simulink model "D_20231120_Modell_Inbetriebnahme_BreakOutBox_Jetson"  (R2022b)
settings: Solver=ode1  StartTime=0.0  StopTime=inf  FixedStep=Ts  RelTol=1e-3
PreLoadFcn:
  | pulsePeriod = 0.05;
  | 
  | Ts = 0.001;
  | 
  | FPGA_Frequency = 75000000;
  | 
  | ts_IO691 = 5e-3;
PostLoadFcn:
  | ewolfSetUp
InitFcn:
  | pulsePeriod = 0.05;
  | 
  | Ts = 0.001;
  | 
  | FPGA_Frequency = 75000000;
  | 
  | ts_IO691 = 5e-3;
StopFcn:
  | Simulink.sdi.clearPreferences;
  | if isfile(['sdi_view_',bdroot,'.mldatx'])
  | Simulink.sdi.view;
  | pause(3);
  | Simulink.sdi.loadView(['sdi_view_',bdroot,]);
  | end
model workspace (MAT data in the model file):
  MaxDreh = 1
values from neighbouring files (symbols this model uses):
  max_ac = 2    [ewolfSetUp.m]
  min_ac = -3    [ewolfSetUp.m]
  PredictionHorizon = 30    [ewolfSetUp.m]
undefined symbols (not defined in the file or in its folder): canChannel, DiscIntNeverNeededParam, Ended, HS, IO291, IO397, max_steer_car, min_steer_car, sigbuilder_block, Single
libraries: lllalib x255, canmsglib x146, simulink x42, speedgoatlib_IO191 x5, speedgoatlib_IO291 x5, slrealtimeiplib x3, speedgoatlib_IO691 x3, slrealtimeutilitieslib x2, spsEdgeDetectorLib x1, simulink_extras x1, speedgoatlib_fpga_dio x1, speedgoatlib_fpga_quadrature x1
(part 1 of 8)
settings Model: SimulationMode=external  ExtModeEnableFloating=off  Creator=daniel.carretero  LastModifiedBy=admin
settings SolverCC: ConcurrentTasks=on  PositivePriorityOrder=on  AutoInsertRateTranBlk=on
settings DataIOCC: ReturnWorkspaceOutputs=off
settings OptimizationCC: BlockReduction=off  OptimizeBlockIOStorage=off
settings DebuggingCC: TasksWithSamePriorityMsg=none  ParameterPrecisionLossMsg=none
settings HardwareCC: ProdBitPerLong=64  ProdLongLongMode=on  ProdHWDeviceType=Intel->x86-64 (Linux 64)
settings ModelReferenceCC: EnableRefExpFcnMdlSchedulingChecks=on
settings RTWCC: Description=Simulink Real-Time  SystemTargetFile=slrealtime.tlc  TemplateMakefile=slrealtime_default_tmf  RTWVerbose=off  Toolchain=Simulink Real-Time Toolchain  BuildConfiguration=Faster Runs  CodeExecutionProfiling=on  TargetLang=C++  DLArmComputeVersion=19.05

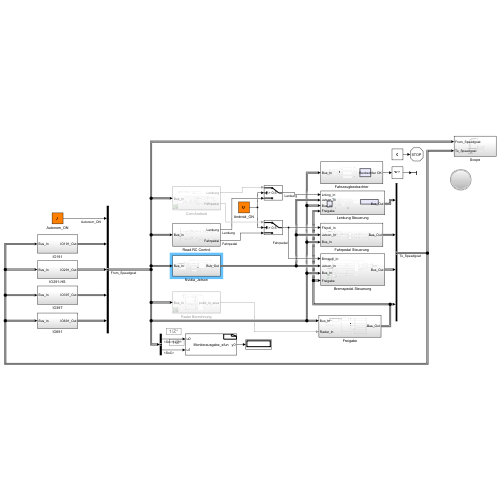
[thumbnail: Simulink's stored preview of the top-level diagram]
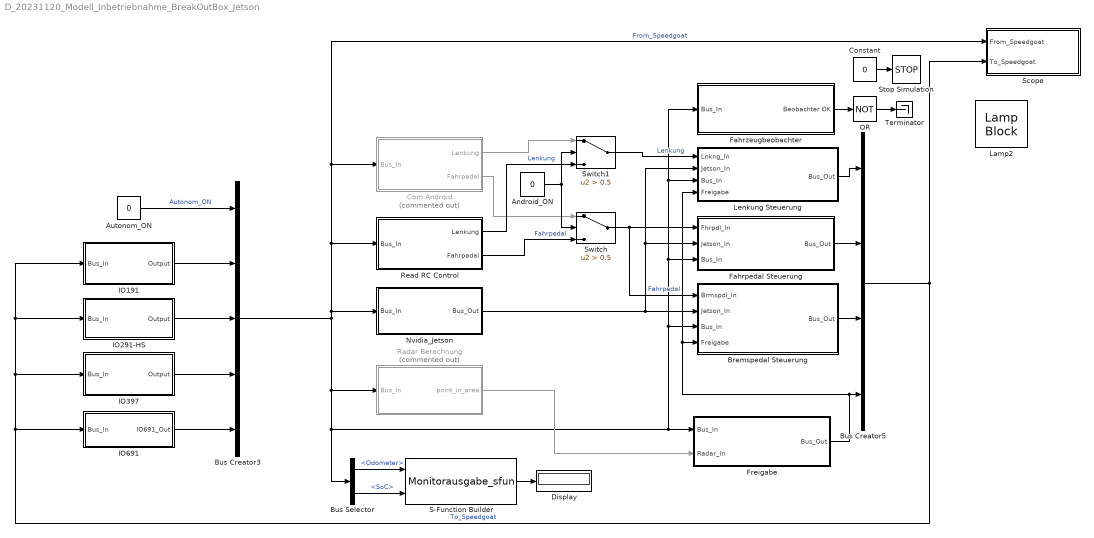
== system D_20231120_Modell_Inbetriebnahme_BreakOutBox_Jetson ==
  Android_ON : Constant  Value=0
  Autonom_ON : Constant  Value=0
  Bremspedal Steuerung : Subsystem
  Bus Creator3 : BusCreator  Inputs=5
  Bus Creator5 : BusCreator  Inputs=4
  Bus Selector : BusSelector  OutputSignals=IO691_Out.IO691_CAN_eWolf.Odometer,IO691_Out.IO691_CAN_eWolf.SoC
  Com Android : Subsystem  Commented=on
  Constant : Constant  Value=0
  Display : Display
  Fahrpedal Steuerung : Subsystem
  Fahrzeugbeobachter : Subsystem
  Freigabe : Subsystem
  IO191 : Subsystem
  IO291-HS : Subsystem
  IO397 : Subsystem
  IO691 : Subsystem
  Lamp2 : LampBlock  LabelPosition=Hide
  Lenkung Steuerung : Subsystem
  Nvidia_Jetson : Subsystem
  OR : Logic  Operator=NOT  AllPortsSameDT=off  OutDataTypeStr=boolean
  Radar Berechnung : Subsystem  Description=|  Commented=on
      | Extract radar data from CAN messages and create vector object with: 1788 fields:
      | 
      | 1. Timestamp
      | 2. cycle_count
      | 3. number of Objects
      | 4. radar timestamp_header
      | 5. CAN ID
      | +++++++++++++++++++++
      | % last point
      | 6. range
      | 7. az
      | 8. vr
      | 9. rcs
      | 10. el
      | ----------------------------------
      | % last point -1
      | 11. range
      | 12. az
      | 13. vr
      | 14. rcs
      | 15. el
      |  ...
      | 
      | empty points, all values == 0
  Read RC Control : Subsystem
  S-Function Builder : S-Function  FunctionName=Monitorausgabe_sfun  SFunctionModules=Monitorausgabe_sfun_wrapper.cpp  SFunctionDeploymentMode=off  EnableBusSupport=off  mask(S-Function Builder){}
      mask help: Simulink:masks:SFunctionBuilder_MD
      mask init:
      | val = [[.9  0.75 0.75 1 1 .9 .9 1]',[1 1 0.75 0.75 .9 .9 1 .9]'];try , sys = get_param(gcb,'SfunBuilderFcnName');if isempty(sys), sys = get_param(gcb,'FunctionName'); end,catch, sys = get_param(gcb,'FunctionName'); end
      settings: CopyFcn=set_param(gcbh,'LinkStatus','none')  OpenFcn=sfunctionwizard(gcbh)
      mask Display: plot(val(:,1),val(:,2)),disp(sys),port_label('input',1,'u0'),port_label('input',2,'u1'),port_label('output',1,'y0')
  Scope : Subsystem
  Stop Simulation : Stop
  Switch : Switch  Criteria=u2 > Threshold  Threshold=0.5  SaturateOnIntegerOverflow=off  InputSameDT=off
  Switch1 : Switch  Criteria=u2 > Threshold  Threshold=0.5  SaturateOnIntegerOverflow=off  InputSameDT=off
  Terminator : Terminator
  wires:
  IO191/1(Output) -> Bus Creator3/2
  IO291-HS/1(Output) -> Bus Creator3/3
  IO397/1(Output) -> Bus Creator3/4
  Bus Creator3/1 -> Scope/1(From_Speedgoat), Com Android/1(Bus_In), Read RC Control/1(Bus_In), Nvidia_Jetson/1(Bus_In), Radar Berechnung/1(Bus_In), Bus Selector/1, Bremspedal Steuerung/3(Bus_In), Fahrzeugbeobachter/1(Bus_In), Lenkung Steuerung/3(Bus_In), Fahrpedal Steuerung/3(Bus_In), Freigabe/1(Bus_In)  "From_Speedgoat"
  Switch/1 -> Bremspedal Steuerung/1(Brmspdl_In), Fahrpedal Steuerung/1(Fhrpdl_In)  "Fahrpedal"
  IO691/1(IO691_Out) -> Bus Creator3/5
  Fahrpedal Steuerung/1(Bus_Out) -> Bus Creator5/2
  Freigabe/1(Bus_Out) -> Bus Creator5/4, Lenkung Steuerung/4(Freigabe), Bremspedal Steuerung/4(Freigabe)
  Bremspedal Steuerung/1(Bus_Out) -> Bus Creator5/3
  Bus Creator5/1 -> IO191/1(Bus_In), IO291-HS/1(Bus_In), IO397/1(Bus_In), IO691/1(Bus_In), Scope/2(To_Speedgoat)  "To_Speedgoat"
  Nvidia_Jetson/1(Bus_Out) -> Bremspedal Steuerung/2(Jetson_In), Lenkung Steuerung/2(Jetson_In), Fahrpedal Steuerung/2(Jetson_In)
  Autonom_ON/1 -> Bus Creator3/1  "Autonom_ON"
  Radar Berechnung/1(point_in_area) -> Freigabe/2(Radar_In)
  Bus Selector/1 -> S-Function Builder/1  "<Odometer>"
  S-Function Builder/1 -> Display/1
  Bus Selector/2 -> S-Function Builder/2  "<SoC>"
  Com Android/1(Lenkung) -> Switch1/1
  Com Android/2(Fahrpedal) -> Switch/1
  Read RC Control/1(Lenkung) -> Switch1/3  "Lenkung"
  Read RC Control/2(Fahrpedal) -> Switch/3  "Fahrpedal"
  Android_ON/1 -> Switch1/2, Switch/2
  Constant/1 -> Stop Simulation/1
  Fahrzeugbeobachter/1(Beobachter OK) -> OR/1
  OR/1 -> Terminator/1
  Switch1/1 -> Lenkung Steuerung/1(Lnkng_In)  "Lenkung"
  Lenkung Steuerung/1(Bus_Out) -> Bus Creator5/1

== system D_20231120_Modell_Inbetriebnahme_BreakOutBox_Jetson/Bremspedal Steuerung ==
  Brmspdl_In : Inport
  Jetson_In : Inport  Port=2
  Bus_In : Inport  Port=3
  Freigabe : Inport  Port=4
  1-D Lookup Table2 : Lookup_n-D  NumberOfTableDimensions=1  BreakpointsForDimension1=[min_ac max_ac]  Table=[-1 1]  InternalRulePriority=Speed  RndMeth=Simplest
  AND3 : Logic  AllPortsSameDT=off  OutDataTypeStr=boolean
  AND4 : Logic  AllPortsSameDT=off  OutDataTypeStr=boolean
  Bus Creator : BusCreator  Inputs=2
  Bus Selector : BusSelector  OutputSignals=IO397_Out.IO397_DIO.IO397_DI_Ch8_Bremsaktuator_Hall_1,IO397_Out.IO397_DIO.IO397_DI_Ch9_Bremsaktuator_Hall_2,IO291_Out.IO291_Iso_DI.IO291_DI_CH3_Brmslcht,IO397_Out.IO397_QAD.IO397_QAD_Turns,Autonom_ON
  Bus Selector1 : BusSelector  OutputSignals=acceleration
  Bus Selector2 : BusSelector  OutputSignals=Taster_Freigabe
  Gain -1 : Gain  Gain=-1
  Moving Average : Subsystem
  Moving Average1 : Subsystem
  QAD Steuerung : Subsystem  Commented=on
  QAD Steuerung1 : Subsystem
  Saturation3 : Saturate  UpperLimit=0  LowerLimit=-1
  Switch : Switch  Criteria=u2 > Threshold  Threshold=0.5  SaturateOnIntegerOverflow=off  InputSameDT=off
  Bus_Out : Outport
  wires:
  Brmspdl_In/1 -> Switch/3
  Saturation3/1 -> Gain -1/1
  Bus_In/1 -> Bus Selector/1
  AND3/1 -> Bus Creator/1  "Bremsaktuator_1"
  AND4/1 -> Bus Creator/2  "Bremsaktuator_2"
  Bus Selector/4 -> QAD Steuerung/1(<QAD_Turns>)  "<IO397_QAD_Turns>"
  Gain -1/1 -> QAD Steuerung1/4(Brk), QAD Steuerung/2(u)  "Bremssignal"
  Bus Selector/1 -> Moving Average/1(In)  "<IO397_DI_Ch8_Bremsaktuator_Hall_1>"
  Bus Selector/2 -> Moving Average1/1(In)  "<IO397_DI_Ch9_Bremsaktuator_Hall_2>"
  Moving Average/1(Hall_A) -> QAD Steuerung1/1(Hall_A)  "Hall_A"
  Moving Average1/1(Hall_B) -> QAD Steuerung1/2(Hall_B)  "Hall_B"
  QAD Steuerung1/1(Rel_1) -> AND3/2  "Rel_1"
  QAD Steuerung1/2(Rel_2) -> AND4/2  "Rel_2"
  Bus Creator/1 -> Bus_Out/1  "Brmskttr"
  Jetson_In/1 -> Bus Selector1/1
  Bus Selector1/1 -> 1-D Lookup Table2/1  "<acceleration>"
  Bus Selector/5 -> Switch/2  "<Autonom_ON>"
  Switch/1 -> Saturation3/1
  1-D Lookup Table2/1 -> Switch/1
  Bus Selector/3 -> QAD Steuerung1/3(BrkPdlSwtch)  "<IO291_DI_CH3_Brmslcht>"
  Freigabe/1 -> Bus Selector2/1
  Bus Selector2/1 -> AND4/1, AND3/1  "<Taster_Freigabe>"

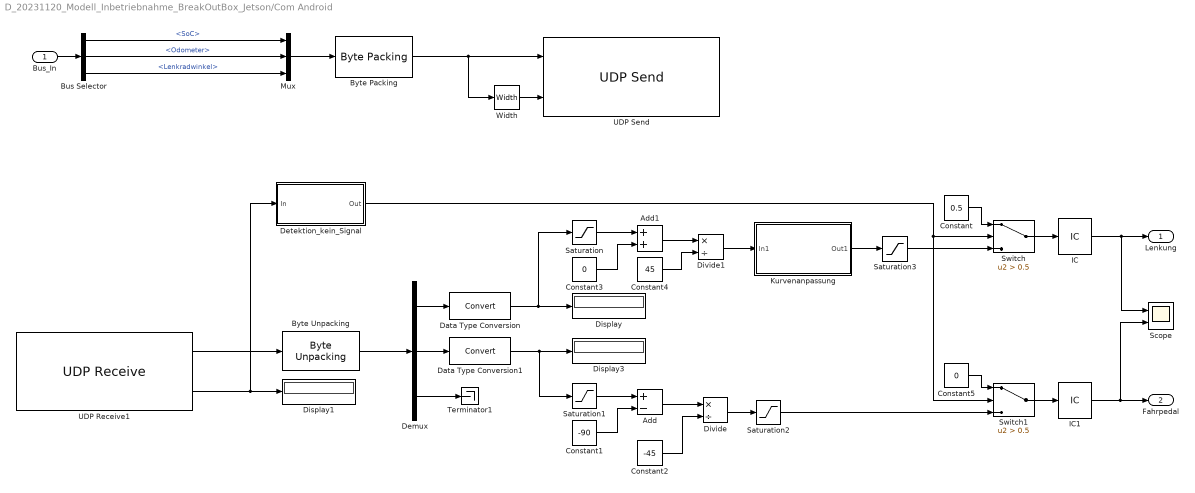
== system D_20231120_Modell_Inbetriebnahme_BreakOutBox_Jetson/Com Android ==
  Bus_In : Inport
  Add : Sum  Inputs=+-
  Add1 : Sum
  Bus Selector : BusSelector  OutputSignals=IO691_Out.IO691_CAN_eWolf.SoC,IO691_Out.IO691_CAN_eWolf.Odometer,IO691_Out.IO691_CAN_Sensoren.Lenkradwinkel
  Byte Packing : slrealtimeutilitieslib/Byte Packing  MaskPackedDataType=uint8  MaskUnpackedDataTypes={'double'}  MaskAlignment=1
  Byte Unpacking : slrealtimeutilitieslib/Byte Unpacking  MaskUnpackedDataTypes={'single'}  MaskUnpackedDataSizes={[3]}  MaskAlignment=1
  Constant : Constant  Value=0.5
  Constant1 : Constant  Value=-90
  Constant2 : Constant  Value=-45
  Constant3 : Constant  Value=0
  Constant4 : Constant  Value=45
  Constant5 : Constant  Value=0
  Data Type Conversion : DataTypeConversion  SaturateOnIntegerOverflow=off  RndMeth=Floor
  Data Type Conversion1 : DataTypeConversion  SaturateOnIntegerOverflow=off  RndMeth=Floor
  Demux : Demux  Outputs=3
  Detektion_kein_Signal : Subsystem
  Display : Display
  Display1 : Display
  Display3 : Display
  Divide : Product  Inputs=*/
  Divide1 : Product  Inputs=*/
  IC : InitialCondition  Value=0.5
  IC1 : InitialCondition  Value=0
  Kurvenanpassung : Subsystem
  Mux : Mux  Inputs=3
  Saturation : Saturate  UpperLimit=45  LowerLimit=-45
  Saturation1 : Saturate  UpperLimit=-45  LowerLimit=-135
  Saturation2 : Saturate  UpperLimit=1  LowerLimit=-1
  Saturation3 : Saturate  UpperLimit=1  LowerLimit=-1
  Scope : Scope  NumInputPorts=2
  Switch : Switch  Criteria=u2 > Threshold  Threshold=0.5  SaturateOnIntegerOverflow=off  InputSameDT=off
  Switch1 : Switch  Criteria=u2 > Threshold  Threshold=0.5  SaturateOnIntegerOverflow=off  InputSameDT=off
  Terminator1 : Terminator
  UDP Receive1 : slrealtimeiplib/UDP Receive  useHostTargetConn=off  ipAddress=192.168.9.10  localPort=25001  rcvWidth=12  rcvFmAny=on  fmAddress='10.10.10.10'  sampleTime=0.001  enableMessage=off  maxPackets=1
  UDP Send : slrealtimeiplib/UDP Send  useHostTargetConn=off  toAddress='192.168.9.255'  toPort=25000  sampleTime=0.1  enableMessage=off  ipAddress=192.168.9.10  localPort=25000
  Width : Width
  Lenkung : Outport
  Fahrpedal : Outport  Port=2
  wires:
  Demux/2 -> Data Type Conversion1/1
  Width/1 -> UDP Send/2
  Byte Unpacking/1 -> Demux/1
  Byte Packing/1 -> Width/1, UDP Send/1
  Bus Selector/2 -> Mux/2  "<Odometer>"
  UDP Receive1/1 -> Byte Unpacking/1
  Mux/1 -> Byte Packing/1
  Demux/3 -> Terminator1/1
  Bus Selector/1 -> Mux/1  "<SoC>"
  Demux/1 -> Data Type Conversion/1
  UDP Receive1/2 -> Detektion_kein_Signal/1(In), Display1/1
  Data Type Conversion1/1 -> Saturation1/1, Display3/1
  Data Type Conversion/1 -> Saturation/1, Display/1
  Bus_In/1 -> Bus Selector/1
  Bus Selector/3 -> Mux/3  "<Lenkradwinkel>"
  Saturation1/1 -> Add/1
  Constant1/1 -> Add/2
  Add/1 -> Divide/1
  Constant2/1 -> Divide/2
  Divide/1 -> Saturation2/1
  Saturation2/1 -> Switch1/3
  Saturation/1 -> Add1/1
  Constant3/1 -> Add1/2
  Add1/1 -> Divide1/1
  Constant4/1 -> Divide1/2
  IC/1 -> Scope/1, Lenkung/1
  IC1/1 -> Scope/2, Fahrpedal/1
  Divide1/1 -> Kurvenanpassung/1(In1)
  Switch/1 -> IC/1
  Switch1/1 -> IC1/1
  Detektion_kein_Signal/1(Out) -> Switch1/2, Switch/2
  Constant/1 -> Switch/1
  Constant5/1 -> Switch1/1
  Saturation3/1 -> Switch/3
  Kurvenanpassung/1(Out1) -> Saturation3/1

== system D_20231120_Modell_Inbetriebnahme_BreakOutBox_Jetson/Fahrpedal Steuerung ==
  Fhrpdl_In : Inport
  Jetson_In : Inport  Port=2
  Bus_In : Inport  Port=3
  1-D Lookup Table : Lookup_n-D  NumberOfTableDimensions=1  BreakpointsForDimension1=[0:1]  Table=[0.8 4.8]  InternalRulePriority=Speed  RndMeth=Simplest
  1-D Lookup Table1 : Lookup_n-D  NumberOfTableDimensions=1  BreakpointsForDimension1=[0:1]  Table=[0.4 2.4]  InternalRulePriority=Speed  RndMeth=Simplest
  1-D Lookup Table2 : Lookup_n-D  NumberOfTableDimensions=1  BreakpointsForDimension1=[min_ac max_ac]  Table=[-1 1]  InternalRulePriority=Speed  RndMeth=Simplest
  Bias1 : Bias  SaturateOnIntegerOverflow=off
  Bias2 : Bias  SaturateOnIntegerOverflow=off
  Bus Creator : BusCreator  Inputs=2
  Bus Selector : BusSelector  OutputSignals=acceleration
  Bus Selector1 : BusSelector  OutputSignals=Autonom_ON
  IC2 : InitialCondition  Value=0.8
  IC3 : InitialCondition  Value=0.4
  Saturation3 : Saturate  UpperLimit=1  LowerLimit=0
  Switch : Switch  Criteria=u2 > Threshold  Threshold=0.5  SaturateOnIntegerOverflow=off  InputSameDT=off
  Bus_Out : Outport
  wires:
  Bias1/1 -> Bus Creator/1  "Ausgabe_Gaspedal_FP_1_G"
  Bias2/1 -> Bus Creator/2  "Ausgabe_Gaspedal_FP_2_G"
  IC2/1 -> Bias1/1
  IC3/1 -> Bias2/1
  1-D Lookup Table/1 -> IC2/1
  Saturation3/1 -> 1-D Lookup Table1/1, 1-D Lookup Table/1
  1-D Lookup Table1/1 -> IC3/1
  Bus Creator/1 -> Bus_Out/1  "Fhrpdl"
  Jetson_In/1 -> Bus Selector/1
  Bus Selector/1 -> 1-D Lookup Table2/1  "<acceleration>"
  Bus_In/1 -> Bus Selector1/1
  Bus Selector1/1 -> Switch/2  "<Autonom_ON>"
  Fhrpdl_In/1 -> Switch/3
  Switch/1 -> Saturation3/1
  1-D Lookup Table2/1 -> Switch/1

== system D_20231120_Modell_Inbetriebnahme_BreakOutBox_Jetson/Fahrzeugbeobachter ==
  note: Aukustische und optische Übergabe
      | an Fahrer
  Bus_In : Inport
  AND : Logic  Inputs=3  AllPortsSameDT=off  OutDataTypeStr=boolean
  Bus Selector : BusSelector  OutputSignals=IO691_Out.IO691_CAN_Sensoren.Lenkradwinkel,IO691_Out.IO691_CAN_eWolf.CarSpeed,IO691_Out.IO691_CAN_Sensoren.Gierrate,IO691_Out.IO691_CAN_Sensoren.Gierbeschleunigung,IO691_Out.IO691_CAN_Sensoren.AY,IO691_Out.IO691_CAN_Sensoren.AX
  Constant3 : Constant  Value=10
  Derivative : Derivative
  Fahrzeuggeschwindigkeit : MATLAB Function  TreatAsAtomicUnit=on
  IC2 : InitialCondition
  Lamp{1..4} (4 alike) : LampBlock  LabelPosition=Hide
  Lenkradwinkel : MATLAB Function  TreatAsAtomicUnit=on
  Lenkradwinkelgeschwindigkeit : MATLAB Function  TreatAsAtomicUnit=on
  Product : Product
  Terminator3 : Terminator  Commented=on
  Terminator4 : Terminator
  Terminator5 : Terminator  Commented=on
  Terminator6 : Terminator  Commented=on
  Beobachter OK : Outport
  wires:
  Bus_In/1 -> Bus Selector/1
  Bus Selector/3 -> Terminator4/1  "<Gierrate>"
  Bus Selector/4 -> Terminator3/1  "<Gierbeschleunigung>"
  Bus Selector/6 -> Terminator6/1  "<AX>"
  Bus Selector/5 -> Terminator5/1  "<AY>"
  Bus Selector/1 -> Derivative/1, Lenkradwinkel/2(lenkradwinkel)  "<Lenkradwinkel>"
  Constant3/1 -> Product/2
  Bus Selector/2 -> Product/1  "<CarSpeed>"
  Product/1 -> Lenkradwinkel/1(geschwindigkeitFahrzeug), Fahrzeuggeschwindigkeit/1(geschwindigkeitFahrzeug), Lenkradwinkelgeschwindigkeit/1(geschwindigkeitFahrzeug)
  Derivative/1 -> Lenkradwinkelgeschwindigkeit/2(geschwindigkeitLenkradwinkel)
  Lenkradwinkelgeschwindigkeit/1(geschwindigkeitLenkradwinkel_OK) -> AND/2
  Lenkradwinkel/1(lenkradwinkel_OK) -> AND/1
  Fahrzeuggeschwindigkeit/1(geschwindigkeitFahrzeug_OK) -> AND/3
  AND/1 -> IC2/1
  IC2/1 -> Beobachter OK/1

== system D_20231120_Modell_Inbetriebnahme_BreakOutBox_Jetson/Freigabe ==
  Bus_In : Inport
  Radar_In : Inport  Port=2
  Bus Creator : BusCreator  Inputs=8
  Constant13 : Constant
  Constant8 : Constant  Value=0
  Freigabe : Subsystem
  Gain{4..9} (6 alike) : Gain
  Terminator : Terminator
  Totmann : Subsystem
  Bus_Out : Outport
  wires:
  Totmann/1(Totmann_Freigabe) -> Freigabe/2(Totmann_In)
  Bus_In/1 -> Freigabe/1(Bus_In), Totmann/1(Bus_In)
  Totmann/2(Totmann_LED) -> Gain4/1
  Gain4/1 -> Bus Creator/7  "LED_Totmann"
  Gain8/1 -> Bus Creator/3  "LG_FET_1_On"
  Gain9/1 -> Bus Creator/4  "LG_FET_2_On"
  Gain7/1 -> Bus Creator/2  "FP_FET_2_On"
  Gain5/1 -> Bus Creator/6  "Taster_Freigabe"
  Freigabe/1(Freigabe_Out) -> Gain5/1, Gain9/1, Gain8/1, Gain7/1, Gain6/1
  Constant8/1 -> Bus Creator/5  "Br_Licht_On"
  Gain6/1 -> Bus Creator/1  "FP_FET_1_On"
  Bus Creator/1 -> Bus_Out/1  "Freigabe"
  Constant13/1 -> Bus Creator/8  "USS_Reverse"
  Radar_In/1 -> Terminator/1

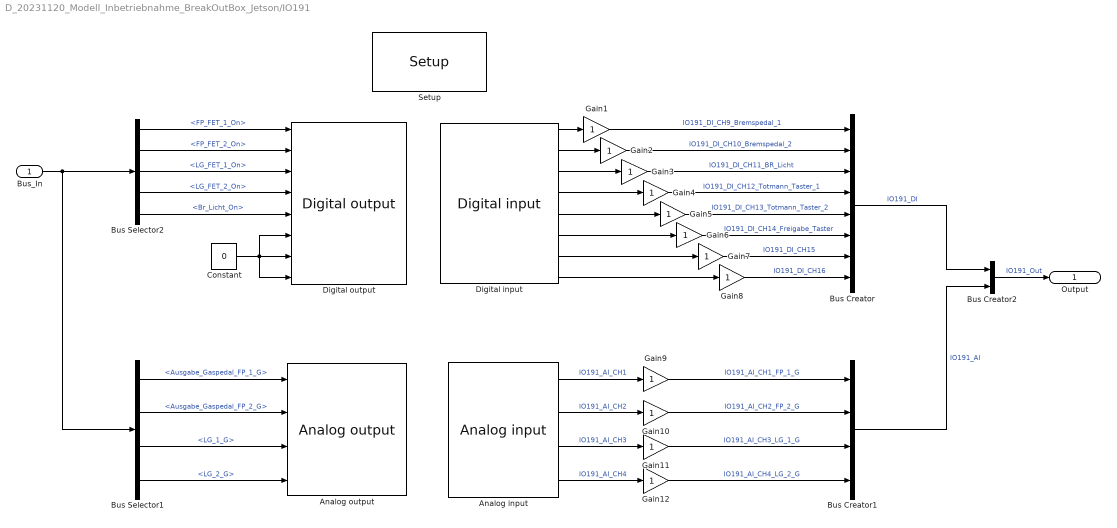
== system D_20231120_Modell_Inbetriebnahme_BreakOutBox_Jetson/IO191 ==
  Bus_In : Inport
  "Analog input " : speedgoatlib_IO191/Analog input   parModuleId=1  parSampleTime=Ts  parPciSlot=-1  parAdcChannels=[1 2 3 4]  parAdcMode=2  parAdcRanges=[4 4 4 4]  parAdcRate=100000  parAdcInitValues=[0 0]  parAdcResets=[1 1]
      settings: SourceProductName=Simulink Real-Time: Speedgoat I/O Blockset
  "Analog output " : speedgoatlib_IO191/Analog output   parModuleId=1  parSampleTime=Ts  parPciSlot=-1  parDacChannels=[1 2 3 4]  parModuleType=1  parDacRanges=[1 1 1 1]  parDacInitValues=[0 0 2.5 2.5]  parDacResets=[1 1 1 1]
      settings: SourceProductName=Simulink Real-Time: Speedgoat I/O Blockset
  Bus Creator : BusCreator  Inputs=8
  Bus Creator1 : BusCreator  Inputs=4
  Bus Creator2 : BusCreator  Inputs=2
  Bus Selector1 : BusSelector  OutputSignals=Fhrpdl.Ausgabe_Gaspedal_FP_1_G,Fhrpdl.Ausgabe_Gaspedal_FP_2_G,Lnkng.LG_1_G,Lnkng.LG_2_G
  Bus Selector2 : BusSelector  OutputSignals=Freigabe.FP_FET_1_On,Freigabe.FP_FET_2_On,Freigabe.LG_FET_1_On,Freigabe.LG_FET_2_On,Freigabe.Br_Licht_On
  Constant : Constant  Value=0
  "Digital input " : speedgoatlib_IO191/Digital input   parModuleId=1  parSampleTime=Ts  parPciSlot=-1  parDiChannels=[9 10 11 12 13 14 15 16]
      settings: SourceProductName=Simulink Real-Time: Speedgoat I/O Blockset
  "Digital output " : speedgoatlib_IO191/Digital output   parModuleId=1  parSampleTime=Ts  parPciSlot=-1  parDoChannels=[1 2 3 4 5 6 7 8]  parDoInitValues=[0 0 0 0 0 0 0 0]  parDoResets=[1 1 1 1 1 1 1 1]
      settings: SourceProductName=Simulink Real-Time: Speedgoat I/O Blockset
  Gain{1..12} (12 alike) : Gain
  "Setup " : speedgoatlib_IO191/Setup   parModuleId=1  parPciSlot=-1  parTriggerSignal=TTL  parAdcChannels=[1 2 3 4]  parAdcRanges=[4 4 4 4]  parAdcChannel1=on  parAdcChannel2=on  parAdcChannel3=on  parAdcChannel4=on  parAdcChannel5=off  parAdcChannel6=off  parAdcChannel7=off  parAdcChannel8=off  parAdcMode=Single-Ended  parAdcRate=100000  parAdcRange11=+-5.12 V  parAdcRange21=+-24.576 V  parAdcRange12=+-5.12 V  parAdcRange22=+-24.576 V  parAdcRange13=+-5.12 V  parAdcRange23=+-24.576 V  parAdcRange14=+-5.12 V  parAdcRange24=+-24.576 V  parAdcRange15=+-10.24 V  parAdcRange25=+-24.576 V  parAdcRange16=+-10.24 V  parAdcRange26=+-24.576 V  parAdcRange17=+-10.24 V  parAdcRange27=+-24.576 V  parAdcRange18=+-10.24 V  parAdcRange28=+-24.576 V  parDacChannels=[1 2 3 4]  parDacChannel1=on  parDacChannel2=on  parDacChannel3=on  parDacChannel4=on  parDacMode=Single-Ended  parDacRanges=[1 1 1 1]  parDacInitValues=[0 0 2.5 2.5]  parDacResets=[1 1 1 1]  parDacRange1=0 V to 5 V  parDacInitValue1=0  parDacReset1=on  parDacRange2=0 V to 5 V  parDacInitValue2=0  parDacReset2=on  parDacRange3=0 V to 5 V  parDacInitValue3=2.5  parDacReset3=on  parDacRange4=0 V to 5 V  parDacInitValue4=2.5  parDacReset4=on  parDiChannels=[9 10 11 12 13 14 15 16]  parDoChannels=[1 2 3 4 5 6 7 8]  parDioFirstControl=1  parDioSecondControl=0  parDioChannel1=Out  parExtra1=I  parExtra2=I  parExtra3=I  parDioChannel2=In  parDioChannel3=In  parDioChannel4=In  parDioChannel5=In  parDioChannel6=In  parDioChannel7=In  parDioChannel8=In  parDioChannel9=In  parDoInitValues=[0 0 0 0]  parDoResets=[1 1 1 1]  parDoInitValue1=0  parDoReset1=on  parDoInitValue2=0  parDoReset2=on  parDoInitValue3=0  parDoReset3=on  parDoInitValue4=0  parDoReset4=on  parDoInitValue5=0  parDoReset5=on  parDoInitValue6=0  parDoReset6=on  parDoInitValue7=0  parDoReset7=on  parDoInitValue8=0  parDoReset8=on  parDoInitValue9=0  parDoReset9=on  parDoInitValue10=0  parDoReset10=on  parDoInitValue11=0  parDoReset11=on  parDoInitValue12=0  parDoReset12=on  parDoInitValue13=0  parDoReset13=on  parDoInitValue14=0  parDoReset14=on  parDoInitValue15=0  parDoReset15=on  parDoInitValue16=0  parDoReset16=on
      settings: SourceProductName=Simulink Real-Time: Speedgoat I/O Blockset
  Output : Outport
  wires:
  "Digital input "/7 -> Gain7/1
  "Digital input "/1 -> Gain1/1
  "Digital input "/6 -> Gain6/1
  "Digital input "/8 -> Gain8/1
  "Digital input "/5 -> Gain5/1
  "Digital input "/4 -> Gain4/1
  "Digital input "/3 -> Gain3/1
  "Digital input "/2 -> Gain2/1
  Gain1/1 -> Bus Creator/1  "IO191_DI_CH9_Bremspedal_1"
  Gain2/1 -> Bus Creator/2  "IO191_DI_CH10_Bremspedal_2"
  Gain3/1 -> Bus Creator/3  "IO191_DI_CH11_BR_Licht"
  Gain4/1 -> Bus Creator/4  "IO191_DI_CH12_Totmann_Taster_1"
  Gain5/1 -> Bus Creator/5  "IO191_DI_CH13_Totmann_Taster_2"
  Gain6/1 -> Bus Creator/6  "IO191_DI_CH14_Freigabe_Taster"
  Gain7/1 -> Bus Creator/7  "IO191_DI_CH15"
  Gain8/1 -> Bus Creator/8  "IO191_DI_CH16"
  "Analog input "/1 -> Gain9/1  "IO191_AI_CH1"
  "Analog input "/2 -> Gain10/1  "IO191_AI_CH2"
  "Analog input "/3 -> Gain11/1  "IO191_AI_CH3"
  "Analog input "/4 -> Gain12/1  "IO191_AI_CH4"
  Bus Creator/1 -> Bus Creator2/1  "IO191_DI"
  Bus Creator1/1 -> Bus Creator2/2  "IO191_AI"
  Bus Creator2/1 -> Output/1  "IO191_Out"
  Gain9/1 -> Bus Creator1/1  "IO191_AI_CH1_FP_1_G"
  Gain10/1 -> Bus Creator1/2  "IO191_AI_CH2_FP_2_G"
  Gain11/1 -> Bus Creator1/3  "IO191_AI_CH3_LG_1_G"
  Gain12/1 -> Bus Creator1/4  "IO191_AI_CH4_LG_2_G"
  Constant/1 -> "Digital output "/6, "Digital output "/8, "Digital output "/7
  Bus_In/1 -> Bus Selector1/1, Bus Selector2/1
  Bus Selector2/1 -> "Digital output "/1  "<FP_FET_1_On>"
  Bus Selector2/2 -> "Digital output "/2  "<FP_FET_2_On>"
  Bus Selector2/3 -> "Digital output "/3  "<LG_FET_1_On>"
  Bus Selector2/4 -> "Digital output "/4  "<LG_FET_2_On>"
  Bus Selector2/5 -> "Digital output "/5  "<Br_Licht_On>"
  Bus Selector1/2 -> "Analog output "/2  "<Ausgabe_Gaspedal_FP_2_G>"
  Bus Selector1/1 -> "Analog output "/1  "<Ausgabe_Gaspedal_FP_1_G>"
  Bus Selector1/3 -> "Analog output "/3  "<LG_1_G>"
  Bus Selector1/4 -> "Analog output "/4  "<LG_2_G>"

== system D_20231120_Modell_Inbetriebnahme_BreakOutBox_Jetson/IO291-HS ==
  Bus_In : Inport
  Alive : Constant  Value=0
  Bus Creator : BusCreator  Inputs=1
  Bus Creator1 : BusCreator  Inputs=3
  Bus Creator2 : BusCreator  Inputs=2
  Bus Selector1 : BusSelector  OutputSignals=Brmskttr.Bremsaktuator_1,Brmskttr.Bremsaktuator_2,Freigabe.USS_Reverse,Freigabe.LED_Totmann,Freigabe.Taster_Freigabe
  Data Type Conversion : DataTypeConversion  SaturateOnIntegerOverflow=off  RndMeth=Floor
  Data Type Conversion1 : DataTypeConversion  SaturateOnIntegerOverflow=off  RndMeth=Floor
  "FET digital output " : speedgoatlib_IO291/FET digital output   parModuleId=1  parSampleTime=Ts  parPciSlot=-1  parFetDoChannels=[1 2 4 5 6]  parFetDoInitValues=[0 0 0 0 0]  parFetDoReset=[1 1 1 1 1]  parModuleType=IO291-HS  parInternalModuleId=1
      settings: SourceProductName=Simulink Real-Time: Speedgoat I/O Blockset
  Gain : Gain
  Gain1 : Gain
  Gain2 : Gain
  "Isolated digital input " : speedgoatlib_IO291/Isolated digital input   parModuleId=1  parSampleTime=Ts  parPciSlot=-1  parIsolDiChannels=[1 2 3]  parModuleType=IO291-HS  parInternalModuleId=1
      settings: SourceProductName=Simulink Real-Time: Speedgoat I/O Blockset
  "LVTTL digital input " : speedgoatlib_IO291/LVTTL digital input   parModuleId=1  parSampleTime=Ts  parPciSlot=-1  parTtlDiChannels=[]  parModuleType=IO291-HS  parInternalModuleId=1
      settings: SourceProductName=Simulink Real-Time: Speedgoat I/O Blockset
  "LVTTL digital output " : speedgoatlib_IO291/LVTTL digital output   parModuleId=1  parSampleTime=Ts  parPciSlot=-1  parTtlDoChannels=[]  parTtlDoInitValues=zeros(1,0)  parTtlDoReset=zeros(1,0)  parModuleType=IO291-HS  parInternalModuleId=1
      settings: SourceProductName=Simulink Real-Time: Speedgoat I/O Blockset
  "Setup " : speedgoatlib_IO291/Setup   parInternalModuleId=1  parPciSlot=-1  parModuleId=1  parModuleType=IO291-HS  parTtlDoChannels=[]  parTtlDoInitValues=0  parTtlDoReset=1  parTtlDiChannels=[]  parIsolDiChannels=[1:3]  parFetDoChannels=[1 2 4:6]  parFetDoInitValues=0  parFetDoReset=1
      settings: SourceProductName=Simulink Real-Time: Speedgoat I/O Blockset
  Output : Outport
  wires:
  "Isolated digital input "/1 -> Gain/1
  "Isolated digital input "/2 -> Gain1/1
  Bus Creator/1 -> Bus Creator2/1  "IO291_LVTTL_DI"
  Bus Creator1/1 -> Bus Creator2/2  "IO291_Iso_DI"
  Bus Creator2/1 -> Output/1  "IO291_Out"
  Alive/1 -> Bus Creator/1  "Alive"
  Data Type Conversion/1 -> "FET digital output "/1
  Data Type Conversion1/1 -> "FET digital output "/2
  Gain/1 -> Bus Creator1/1  "IO291_DI_CH1_NotAus_1"
  Gain1/1 -> Bus Creator1/2  "IO291_DI_CH2_NotAus_2"
  Bus_In/1 -> Bus Selector1/1
  Bus Selector1/1 -> Data Type Conversion/1  "<Bremsaktuator_1>"
  Bus Selector1/2 -> Data Type Conversion1/1  "<Bremsaktuator_2>"
  Bus Selector1/3 -> "FET digital output "/3  "<USS_Reverse>"
  Bus Selector1/4 -> "FET digital output "/4  "<LED_Totmann>"
  Bus Selector1/5 -> "FET digital output "/5  "<Taster_Freigabe>"
  "Isolated digital input "/3 -> Gain2/1
  Gain2/1 -> Bus Creator1/3  "IO291_DI_CH3_Brmslcht"

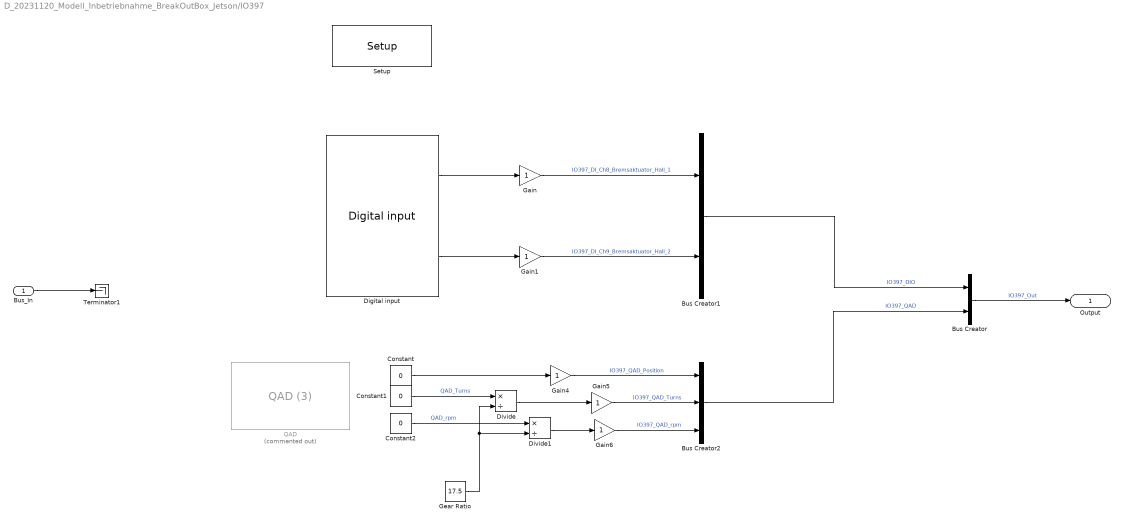
== system D_20231120_Modell_Inbetriebnahme_BreakOutBox_Jetson/IO397 ==
  Bus_In : Inport
  Bus Creator : BusCreator  Inputs=2
  Bus Creator1 : BusCreator  Inputs=2
  Bus Creator2 : BusCreator  Inputs=3
  Constant : Constant  Value=0
  Constant1 : Constant  Value=0
  Constant2 : Constant  Value=0
  Digital input : speedgoatlib_fpga_dio/Digital input  id=1  chan=[8,9]  ts=Ts  pciSlot=-1  board=IO397-50k  vectorizeOutput=off
      settings: SourceProductName=Simulink Real-Time: Speedgoat I/O Blockset
  Divide : Product  Inputs=*/
  Divide1 : Product  Inputs=*/
  Gain{,1,4..6} (5 alike) : Gain
  Gear Ratio : Constant  Value=17.5
  QAD : speedgoatlib_fpga_quadrature/QAD (3)  Commented=on  id=1  board=IO397-50k  chan=1  resetOnStart=on  ts=Ts  pciSlot=-1  operatingMode=Quadrature decoder  indexControlMode=Ignore index  resolution=4x  stepsPerRevolution=12  latchMode=Disabled  interpolatePosition=off  invertAB=off  showClearPositionInput=off  showClearIndexFoundInput=off  showPositionOutput=on  showTurnOutput=on  showSpeedOutput=on  showDirectionOutput=off  showIndexFoundOutput=off
      settings: SourceProductName=Simulink Real-Time: Speedgoat I/O Blockset
  Setup : speedgoatlib_fpga/Setup/Setup  board=IO397-50k  id=1  device_id=1  frontIO=None  rearIO=None  bitstreamFile=speedgoat_IO397_50k_Comms.mat  rev=5.000000  timestamp_string=28/02/23 11:36:55  fpgaFreq=75 MHz  fpgaTick=13.33 ns  ProgSpiFlash=off  ProgBPIFlash=off  pciSlot=-1  PullRPort0=pull-up 3.3V  VioPort0=3.3V  PullRPort1=pull-up 3.3V  VioPort1=3.3V  PullRPort2=pull-up 3.3V  VioPort2=3.3V  PullRPort3=pull-up 3.3V  VioPort3=3.3V  PullRPort4=pull-up 3.3V  VioPort4=3.3V  PullRPort5=pull-up 3.3V  VioPort5=3.3V  PullRPort6=pull-up 3.3V  VioPort6=3.3V  diffLineTermination_rear1=on  diffLineTermination_rear2=on  diffLineTermination_rear3=on  diffLineTermination_rear4=on  diffLineTermination_rear5=on  diffLineTermination_rear6=on  diffLineTermination_rear7=on  diffLineTermination_rear8=on  PullRPort15=pull-down  PullRPort31=pull-up 3.3V  PullRPort47=pull-up 3.3V  PullRPort63=pull-up 3.3V  diffLineTermination_1=on  diffLineTermination_2=on  diffLineTermination_3=on  diffLineTermination_4=on  diffLineTermination_5=on  diffLineTermination_6=on  diffLineTermination_7=on  diffLineTermination_8=on
      settings: SourceProductName=Simulink Real-Time: Speedgoat I/O Blockset
  Terminator1 : Terminator
  Output : Outport
  wires:
  Bus Creator/1 -> Output/1  "IO397_Out"
  Constant/1 -> Gain4/1
  Bus Creator1/1 -> Bus Creator/1  "IO397_DIO"
  Bus Creator2/1 -> Bus Creator/2  "IO397_QAD"
  Divide/1 -> Gain5/1
  Divide1/1 -> Gain6/1
  Gear Ratio/1 -> Divide1/2, Divide/2
  Constant1/1 -> Divide/1  "QAD_Turns"
  Constant2/1 -> Divide1/1  "QAD_rpm"
  Digital input/2 -> Gain1/1
  Digital input/1 -> Gain/1
  Gain/1 -> Bus Creator1/1  "IO397_DI_Ch8_Bremsaktuator_Hall_1"
  Gain1/1 -> Bus Creator1/2  "IO397_DI_Ch9_Bremsaktuator_Hall_2"
  Gain4/1 -> Bus Creator2/1  "IO397_QAD_Position"
  Gain5/1 -> Bus Creator2/2  "IO397_QAD_Turns"
  Gain6/1 -> Bus Creator2/3  "IO397_QAD_rpm"
  Bus_In/1 -> Terminator1/1

== system D_20231120_Modell_Inbetriebnahme_BreakOutBox_Jetson/IO691 ==
  note: PORT 1 - RX
  note: PORT 2 - RX
  Bus_In : Inport
  Bus Creator : BusCreator  Inputs=2
  CAN Read Loop - Port 1 : Subsystem  TreatAsAtomicUnit=on
  CAN Read Loop - Port 3 : Subsystem  TreatAsAtomicUnit=on
  "CAN Setup " : speedgoatlib_IO691/Legacy/CAN Setup   moduletype=IO691  id=1  pciSlot=-1  chn1=CAN (HS)  chn2=CAN (HS)  chn3=Disabled  chn4=Disabled  initStruct=[]  termStruct=[]  ArbitrationbdrChn1=500 kBaud  ArbitrationManbdrChn1=[2,16,63,16]  FdbdrChn1=5.0 MBaud  FdManbdrChn1=[2,2,5,2]  ArbitrationbdrChn2=500 kBaud  ArbitrationManbdrChn2=[2,16,63,16]  FdbdrChn2=5.0 MBaud  FdManbdrChn2=[2,2,5,2]  ArbitrationbdrChn3=1.0 MBaud  ArbitrationManbdrChn3=[2,8,31,8]  FdbdrChn3=5.0 MBaud  FdManbdrChn3=[2,2,5,2]  ArbitrationbdrChn4=1.0 MBaud  ArbitrationManbdrChn4=[2,8,31,8]  FdbdrChn4=5.0 MBaud  FdManbdrChn4=[2,2,5,2]  moduleInitValues=[691 1 -1 -1]
      settings: SourceProductName=Simulink Real-Time: Speedgoat I/O Blockset
  RX Sample Time : Constant  SampleTime=ts_IO691
  Terminator1 : Terminator
  IO691_Out : Outport
  wires:
  RX Sample Time/1 -> CAN Read Loop - Port 3/1(SampleTime), CAN Read Loop - Port 1/1(SampleTime)
  Bus Creator/1 -> IO691_Out/1  "IO691_Out"
  CAN Read Loop - Port 1/1(CAN_Out) -> Bus Creator/2  "IO691_CAN_eWolf"
  CAN Read Loop - Port 3/1(CAN_Out) -> Bus Creator/1  "IO691_CAN_Sensoren"
  Bus_In/1 -> Terminator1/1

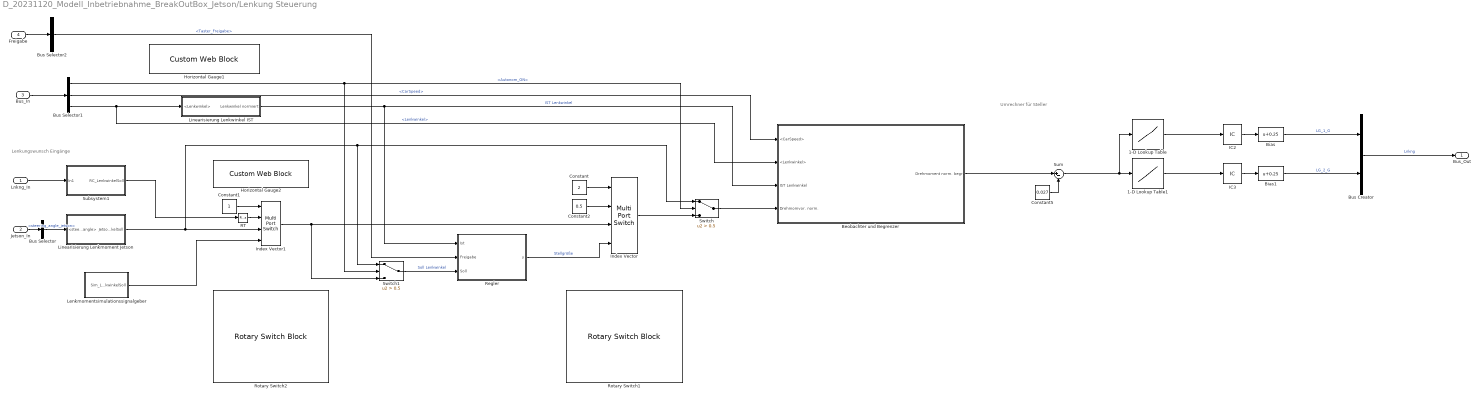
== system D_20231120_Modell_Inbetriebnahme_BreakOutBox_Jetson/Lenkung Steuerung ==
  note: Umrechner für Steller
  note: Lenkungswunsch Eingänge
  Lnkng_In : Inport
  Jetson_In : Inport  Port=2
  Bus_In : Inport  Port=3
  Freigabe : Inport  Port=4
  1-D Lookup Table : Lookup_n-D  NumberOfTableDimensions=1  BreakpointsForDimension1=[0:1]  Table=[1.6 3.4]  InternalRulePriority=Speed  RndMeth=Simplest
  1-D Lookup Table1 : Lookup_n-D  NumberOfTableDimensions=1  BreakpointsForDimension1=[0:1]  Table=[3.4 1.6]  InternalRulePriority=Speed  RndMeth=Simplest
  Beobachter und Begrenzer : Subsystem
  Bias : Bias  Bias=0.25  SaturateOnIntegerOverflow=off
  Bias1 : Bias  Bias=0.25  SaturateOnIntegerOverflow=off
  Bus Creator : BusCreator  Inputs=2
  Bus Selector : BusSelector  OutputSignals=steering_angle_jetson
  Bus Selector1 : BusSelector  OutputSignals=Autonom_ON,IO691_Out.IO691_CAN_eWolf.CarSpeed,IO691_Out.IO691_CAN_Sensoren.Lenkwinkel
  Bus Selector2 : BusSelector  OutputSignals=Taster_Freigabe
  Constant : Constant  Value=2
  Constant1 : Constant
  Constant2 : Constant  Value=0.5
  Constant5 : Constant  Value=0.027
  Horizontal Gauge1 : CustomWebBlock  LabelPosition=Hide  ShowInitialText=on  Configuration="{\"components\":[{\"name\":\"LinearScaleComponent\",\"settings\":{\"bounds\":{\"max\":70,\"min\":0,\"tickInterval\":\"auto\"},\"internalTickHeightScaleFactor\":0.5,\"labelColor\":[255,255,200],\"labelFont\":{\"font\":\"Arial\",\"fontSize\":12},\"labelOffset\":0.05,\"labelTransparency\":1,\"needleImage\":{\"size\":[21,75],\"src\":\"data:image\\/svg+xml;base64,PHN2ZyB4bWxucz0iaHR0cDovL3d3dy53My5vcmcvMjAwMC9zdmciIHhtbG5zOnhsaW5rPSJodHRwOi8vd3d3LnczLm9yZy8xOTk5L3hsaW5rIiB2aWV3Qm94PSIwIDAgMjEgNzUiPjxkZWZzPjxzdHlsZT4uY2xzLTF7ZmlsbDpub25lO30uY2xzLTJ7aXNvbGF0aW9uOmlzb2xhdGU7fS5jbHMtM3tjbGlwLXBhdGg6dXJsKCNjbGlwLXBhdGgpO30uY2xzLTR7b3BhY2l0eTowLjM7bWl4LWJsZW5kLW1vZGU6bXVsdGlwbHk7fS5jbHMtNXtmaWxsOiNlYjI2Mjk7fTwvc3R5bGU+PGNsaXBQYXRoIGlkPSJjbGlwLXBhdGgiIHRyYW5zZm9y ...(+1928 chars)\",\"srcOrientation\":\"Right\"},\"needleOffset\":[0,-0.007413509060955519],\"needleSize\":{\"height\":0.7589285714285714,\"width\":0.11955094537815127},\"position\":[0.09075797872340426,0.019902234636871508,0.9641236033519553,0.7995345744680851],\"referencePoint\":\"auto\",\"scaleColors\":[],\"scaleColorsSize\":0.2,\"scaleDirection\":\"LR\",\"showLabels\":1,\"showMinorTicks\":0,\"showSpanLine\":1,\"showTicks\":1,\"tickColor\":[252,252,197],\"tickTransparency\":1,\"valueBarColor\":[23,89,176],\"valueBarOffset\":0,\"valueBarSize\":0.23,\"valueBarTransparency\":1}},{\"name\":\"BackgroundImageComponent\",\"settings\":{\"image\":{\"size\":[380,101],\"src\":\"data:image\\/svg+xml;base64,PHN2ZyBpZD0iZnJhbWUiIHhtbG5zPSJodHRwOi8vd3d3LnczLm9yZy8yMDAwL3N2ZyIgeG1sbnM6eGxpbms9Imh0dHA6Ly93d3cudzMub3JnLzE5OTkveGxpbmsiIHZpZXdCb3g9IjAgMCAzODAgMTAxIj48ZGVmcz48c3R5bGU+LmNscy0xe2ZpbGw6IzAwMmI0Mjt9LmNscy0ye2ZpbGw6IzQyNzA4Mjt9LmNscy0ze2ZpbGw6dXJsKCNyYWRpYWwtZ3JhZGllbnQpO308L3N0eWxlPjxyYWRpYWxHcmFkaWVudCBpZD0icmFkaWFsLWdyYWRpZW50IiBjeD0iMTkwIiBjeT0iNTAuNSIgcj0iMjY5LjIxIiBncmFkaWVudFVuaXRzPSJ1c2VyU3BhY2VPblVzZSI+PHN0b3Agb2Zmc2V0PSIwLjAxIiBzdG9wLWNvbG9yPSIjM2U0ZjU4Ii8+PHN0b3Agb2Zmc2V0PSIwLjA2IiBzdG9wLWNvbG9yPSIjNDQ1NzYxIi8+PHN0b3Agb2Zmc2V0PSIwLjE1IiBzdG9wLWNvbG9yPSIjNTU2YTc2Ii8+PHN0b3Agb2Zmc2V0PSIwLjI1IiBzdG9wLWNvbG9yPSIjNmQ4ODk1Ii8+PHN0b3Agb2Zmc2V0PSIwLjM4IiBzdG9wLWNvbG9yPSIjOGZiMmMzIi8+PHN0b3Agb2Zmc2V0PSIwLjUyIiBzdG9wLWNvbG9yPSIjYjZlNGZhIi8+PHN0b3Agb2Zmc2V0PSIxIiBzdG9wLWNvbG9yPSIjMTU0NjU3Ii8+PC9yYWRpYWxHcmFkaWVudD48L2RlZnM+PGcgaWQ9IkxheWVyXzIiIGRhdGEtbmFtZT0iTGF5ZXIgMiI+PGcgaWQ9IkxheWVyXzEtMiIgZGF0YS1uYW1lPSJMYXllciAxLTIiPjxyZWN0IGlkPSJyZWN0MTAzNiIgY2xhc3M9ImNscy0xIiB4PSIxMSIgeT0iMTEiIHdpZHRoPSIzNTgiIGhlaWdodD0iNzkiLz48cGF0aCBpZD0icGF0aDEwMzgiIGNsYXNzPSJjbHMtMiIgZD0iTTgsOFY5M0gzNzJWOFpNMzY5LDkwSDExVjExSDM2OVoiLz48cGF0aCBpZD0icGF0aDEwNDAiIGNsYXNzPSJjbHMtMyIgZD0iTTAsMFYxMDFIMzgwVjBaTTM3Miw5M0g4VjhIMzcyWiIvPjwvZz48L2c+PC9zdmc+\",\"srcOrientation\":\"horizontal\"},\"position\":[0,0,1,1],\"scaleMode\":\"0\"}},{\"name\":\"ForegroundImageComponent\",\"settings\":{\"image\":{\"size\":[0,0],\"src\":\"default\",\"srcOrientation\":[]},\"isForeground\":1,\"position\":[0,0,1,1],\"scaleMode\":\"0\"}}],\"settings\":{\"BindingType\":\"signal\",\"backgroundColor\":[0,0,0,\"1\"],\"backgroundOffset\":0,\"backgroundOpacity\":1,\"fixedAspectRatio\":\"on\",\"orientation\":\"horizontal\",\"showBackgroundColor\":false,\"value\":0,\"version\":\"R2022b\"},\"type\":\"LinearGauge\"}"
  Horizontal Gauge2 : CustomWebBlock  LabelPosition=Hide  ShowInitialText=on  Configuration="{\"components\":[{\"name\":\"LinearScaleComponent\",\"settings\":{\"bounds\":{\"max\":1,\"min\":0,\"tickInterval\":0.25},\"internalTickHeightScaleFactor\":0.5,\"labelColor\":[255,255,200],\"labelFont\":{\"font\":\"Arial\",\"fontSize\":12},\"labelOffset\":0.05,\"labelTransparency\":1,\"needleImage\":{\"size\":[21,75],\"src\":\"data:image\\/svg+xml;base64,PHN2ZyB4bWxucz0iaHR0cDovL3d3dy53My5vcmcvMjAwMC9zdmciIHhtbG5zOnhsaW5rPSJodHRwOi8vd3d3LnczLm9yZy8xOTk5L3hsaW5rIiB2aWV3Qm94PSIwIDAgMjEgNzUiPjxkZWZzPjxzdHlsZT4uY2xzLTF7ZmlsbDpub25lO30uY2xzLTJ7aXNvbGF0aW9uOmlzb2xhdGU7fS5jbHMtM3tjbGlwLXBhdGg6dXJsKCNjbGlwLXBhdGgpO30uY2xzLTR7b3BhY2l0eTowLjM7bWl4LWJsZW5kLW1vZGU6bXVsdGlwbHk7fS5jbHMtNXtmaWxsOiNlYjI2Mjk7fTwvc3R5bGU+PGNsaXBQYXRoIGlkPSJjbGlwLXBhdGgiIHRyYW5zZm9y ...(+1928 chars)\",\"srcOrientation\":\"Right\"},\"needleOffset\":[0,-0.007413509060955519],\"needleSize\":{\"height\":0.7589285714285714,\"width\":0.11955094537815127},\"position\":[0.09075797872340426,0.019902234636871508,0.9641236033519553,0.7995345744680851],\"referencePoint\":\"auto\",\"scaleColors\":[],\"scaleColorsSize\":0.2,\"scaleDirection\":\"LR\",\"showLabels\":1,\"showMinorTicks\":0,\"showSpanLine\":1,\"showTicks\":1,\"tickColor\":[252,252,197],\"tickTransparency\":1,\"valueBarColor\":[23,89,176],\"valueBarOffset\":0,\"valueBarSize\":0.23,\"valueBarTransparency\":1}},{\"name\":\"BackgroundImageComponent\",\"settings\":{\"image\":{\"size\":[380,101],\"src\":\"data:image\\/svg+xml;base64,PHN2ZyBpZD0iZnJhbWUiIHhtbG5zPSJodHRwOi8vd3d3LnczLm9yZy8yMDAwL3N2ZyIgeG1sbnM6eGxpbms9Imh0dHA6Ly93d3cudzMub3JnLzE5OTkveGxpbmsiIHZpZXdCb3g9IjAgMCAzODAgMTAxIj48ZGVmcz48c3R5bGU+LmNscy0xe2ZpbGw6IzAwMmI0Mjt9LmNscy0ye2ZpbGw6IzQyNzA4Mjt9LmNscy0ze2ZpbGw6dXJsKCNyYWRpYWwtZ3JhZGllbnQpO308L3N0eWxlPjxyYWRpYWxHcmFkaWVudCBpZD0icmFkaWFsLWdyYWRpZW50IiBjeD0iMTkwIiBjeT0iNTAuNSIgcj0iMjY5LjIxIiBncmFkaWVudFVuaXRzPSJ1c2VyU3BhY2VPblVzZSI+PHN0b3Agb2Zmc2V0PSIwLjAxIiBzdG9wLWNvbG9yPSIjM2U0ZjU4Ii8+PHN0b3Agb2Zmc2V0PSIwLjA2IiBzdG9wLWNvbG9yPSIjNDQ1NzYxIi8+PHN0b3Agb2Zmc2V0PSIwLjE1IiBzdG9wLWNvbG9yPSIjNTU2YTc2Ii8+PHN0b3Agb2Zmc2V0PSIwLjI1IiBzdG9wLWNvbG9yPSIjNmQ4ODk1Ii8+PHN0b3Agb2Zmc2V0PSIwLjM4IiBzdG9wLWNvbG9yPSIjOGZiMmMzIi8+PHN0b3Agb2Zmc2V0PSIwLjUyIiBzdG9wLWNvbG9yPSIjYjZlNGZhIi8+PHN0b3Agb2Zmc2V0PSIxIiBzdG9wLWNvbG9yPSIjMTU0NjU3Ii8+PC9yYWRpYWxHcmFkaWVudD48L2RlZnM+PGcgaWQ9IkxheWVyXzIiIGRhdGEtbmFtZT0iTGF5ZXIgMiI+PGcgaWQ9IkxheWVyXzEtMiIgZGF0YS1uYW1lPSJMYXllciAxLTIiPjxyZWN0IGlkPSJyZWN0MTAzNiIgY2xhc3M9ImNscy0xIiB4PSIxMSIgeT0iMTEiIHdpZHRoPSIzNTgiIGhlaWdodD0iNzkiLz48cGF0aCBpZD0icGF0aDEwMzgiIGNsYXNzPSJjbHMtMiIgZD0iTTgsOFY5M0gzNzJWOFpNMzY5LDkwSDExVjExSDM2OVoiLz48cGF0aCBpZD0icGF0aDEwNDAiIGNsYXNzPSJjbHMtMyIgZD0iTTAsMFYxMDFIMzgwVjBaTTM3Miw5M0g4VjhIMzcyWiIvPjwvZz48L2c+PC9zdmc+\",\"srcOrientation\":\"horizontal\"},\"position\":[0,0,1,1],\"scaleMode\":\"0\"}},{\"name\":\"ForegroundImageComponent\",\"settings\":{\"image\":{\"size\":[0,0],\"src\":\"default\",\"srcOrientation\":[]},\"isForeground\":1,\"position\":[0,0,1,1],\"scaleMode\":\"0\"}}],\"settings\":{\"BindingType\":\"signal\",\"backgroundColor\":[0,0,0,\"1\"],\"backgroundOffset\":0,\"backgroundOpacity\":1,\"fixedAspectRatio\":\"on\",\"orientation\":\"horizontal\",\"showBackgroundColor\":false,\"value\":0,\"version\":\"R2022b\"},\"type\":\"LinearGauge\"}"
  IC2 : InitialCondition  Value=2.5
  IC3 : InitialCondition  Value=2.5
  Index Vector : MultiPortSwitch  DataPortOrder=Zero-based contiguous  zeroidx=on  SaturateOnIntegerOverflow=off  InputSameDT=off
  Index Vector1 : MultiPortSwitch  DataPortOrder=Zero-based contiguous  zeroidx=on  SaturateOnIntegerOverflow=off  InputSameDT=off
  Lenkmomentsimulationssignalgeber : Subsystem
  Linearisierung Lenkmoment Jetson : Subsystem
  Linearisierung Lenkwinkel IST : Subsystem
  RT : RateTransition  OutPortSampleTime=0.001
  Regler : Subsystem
  Rotary Switch1 : RotarySwitchBlock
      settings: Values={{'AUS', 'Direkt', 'Regler'}, [0 1 2]}
  Rotary Switch2 : RotarySwitchBlock
      settings: Values={{'RC', 'Jetson', 'Simulation'}, [0 1 2]}
  Subsystem1 : Subsystem
  Sum : Sum  Inputs=|+-
  Switch : Switch  Criteria=u2 > Threshold  Threshold=0.5  SaturateOnIntegerOverflow=off  InputSameDT=off
  Switch1 : Switch  Criteria=u2 > Threshold  Threshold=0.5  SaturateOnIntegerOverflow=off  InputSameDT=off
  Bus_Out : Outport
  wires:
  Index Vector/1 -> Switch/3
  Constant2/1 -> Index Vector/2
  Constant/1 -> Index Vector/1
  Index Vector1/1 -> Index Vector/3, Switch1/3
  Bus Creator/1 -> Bus_Out/1  "Lnkng"
  Bus Selector1/1 -> Switch/2, Switch1/2  "<Autonom_ON>"
  Switch1/1 -> Regler/3(Soll)  "Soll Lenkwinkel"
  Constant5/1 -> Sum/2
  Jetson_In/1 -> Bus Selector/1
  Constant1/1 -> Index Vector1/1
  RT/1 -> Index Vector1/2
  Bus Selector/1 -> Linearisierung Lenkmoment Jetson/1(<steering_angle>)  "<steering_angle_jetson>"
  Linearisierung Lenkwinkel IST/1(Lenkwinkel normiert) -> Regler/1("Ist "), Beobachter und Begrenzer/3(IST Lenkwinkel)  "IST Lenkwinkel"
  Regler/1(y) -> Index Vector/4  "Stellgröße"
  Bus Selector1/3 -> Beobachter und Begrenzer/2(<Lenkwinkel>), Linearisierung Lenkwinkel IST/1(<Lenkwinkel>)  "<Lenkwinkel>"
  Freigabe/1 -> Bus Selector2/1
  Bus Selector2/1 -> Regler/2(Freigabe)  "<Taster_Freigabe>"
  Bus Selector1/2 -> Beobachter und Begrenzer/1(<CarSpeed>)  "<CarSpeed>"
  Switch/1 -> Beobachter und Begrenzer/4(Drehmomvor. norm.)
  Lnkng_In/1 -> Subsystem1/1(In1)
  Subsystem1/1(RC_LenkwinkelSoll) -> RT/1
  Bias/1 -> Bus Creator/1  "LG_1_G"
  Sum/1 -> 1-D Lookup Table/1, 1-D Lookup Table1/1
  1-D Lookup Table1/1 -> IC3/1
  1-D Lookup Table/1 -> IC2/1
  IC2/1 -> Bias/1
  IC3/1 -> Bias1/1
  Bias1/1 -> Bus Creator/2  "LG_2_G"
  Bus_In/1 -> Bus Selector1/1
  Beobachter und Begrenzer/1(Drehmoment norm. begr.) -> Sum/1
  Lenkmomentsimulationssignalgeber/1(Sim_LenkwinkelSoll) -> Index Vector1/4
  Linearisierung Lenkmoment Jetson/1(Jetson_LenkwinkelSoll) -> Index Vector1/3, Switch1/1, Switch/1

== system D_20231120_Modell_Inbetriebnahme_BreakOutBox_Jetson/Nvidia_Jetson ==
  Bus_In : Inport
  Bus Creator : BusCreator  Inputs=2
  Bus Selector1 : BusSelector  OutputSignals=IO691_Out.IO691_CAN_Sensoren.Radar.radar data (length 1788),IO691_Out.IO691_CAN_Sensoren.Lenkradwinkel,IO691_Out.IO691_CAN_eWolf.CarSpeed
  Data Type Conversion : DataTypeConversion  SaturateOnIntegerOverflow=off  RndMeth=Floor
  Display : Display
  From Jetson : slrealtimeiplib/UDP Receive  useHostTargetConn=off  ipAddress=10.42.0.10  localPort=5500  rcvWidth=56  rcvFmAny=on  fmAddress=10.10.10.10  sampleTime=-1  enableMessage=off  maxPackets=1
  LaneFollowingAndControl : Subsystem
  PackLaneBus : MATLABSystem  System=packLaneMarkerBus  Camera=camera  SimulateUsing=Code generation
      mask Type: packLaneMarkerBus
      mask Display:
      | disp('packLaneMarkerBus');
      | port_label('input',1,'msgs');
      | port_label('output',1,'lanes');
  Rate Transition1 : RateTransition
  Rate Transition2 : RateTransition
  Set Velocity : Constant  Value=5  OutDataTypeStr=single
  Terminator{,1..3} (4 alike) : Terminator
  steering_accel : MATLAB Function  TreatAsAtomicUnit=on
  Bus_Out : Outport
  wires:
  Bus Selector1/3 -> Rate Transition1/1  "<CarSpeed>"
  LaneFollowingAndControl/2(acceleration) -> Bus Creator/2  "acceleration"
  Rate Transition2/1 -> Terminator/1  "Lenkwinkel"
  Rate Transition1/1 -> LaneFollowingAndControl/2(Longitudinal_Velocity)  "Longitudinal_Velocity"
  Bus_In/1 -> Bus Selector1/1
  LaneFollowingAndControl/1(steering_angle) -> Terminator2/1  "steering_angle_speedgoat"
  From Jetson/2 -> Terminator3/1
  Bus Selector1/2 -> Rate Transition2/1  "<Lenkradwinkel>"
  From Jetson/1 -> steering_accel/1(msgs), PackLaneBus/1
  PackLaneBus/1 -> LaneFollowingAndControl/3(Lane Detections)
  Set Velocity/1 -> LaneFollowingAndControl/1(Set velocity)
  Bus Creator/1 -> Bus_Out/1  "Nvidia_Jetson"
  Bus Selector1/1 -> Data Type Conversion/1  "<radar data (length 1788)>"
  Data Type Conversion/1 -> Terminator1/1  "Radar_Data"
  steering_accel/1(steering_angle) -> Bus Creator/1, Display/1  "steering_angle_jetson"

== system D_20231120_Modell_Inbetriebnahme_BreakOutBox_Jetson/Radar Berechnung ==
  Bus_In : Inport
  Add : Sum
  Add1 : Sum
  Bus Selector : BusSelector  OutputSignals=IO691_Out.IO691_CAN_Sensoren.Radar.Radar_Mode,IO691_Out.IO691_CAN_eWolf.CarSpeed,IO691_Out.IO691_CAN_Sensoren.Radar.Radar_Punkt
  Constant : Constant  Value=10
  Divide : Product  Inputs=*/
  Product : Product
  azimuth_max : Constant  Value=5
  azimuth_min : Constant  Value=-5
  current_ego_wheel_angle : Constant  Value=0
  elevation_max : Constant
  elevation_min : Constant  Value=-1
  range_min : Constant  Value=0
  range_savety_const : Constant  Value=2
  rcs_max : Constant  Value=100
  rcs_min : Constant  Value=0
  speed_min : Constant  Value=0
  sub_point_in_area : Subsystem  TreatAsAtomicUnit=on
  point_in_area : Outport
  wires:
  sub_point_in_area/1(Output) -> point_in_area/1
  rcs_max/1 -> sub_point_in_area/8(rcs_max)
  rcs_min/1 -> sub_point_in_area/7(rcs_min)
  elevation_max/1 -> sub_point_in_area/10(elevation_max)
  elevation_min/1 -> sub_point_in_area/9(elevation_min)
  Bus Selector/2 -> Divide/1, sub_point_in_area/6(speed_max)  "<CarSpeed>"
  speed_min/1 -> sub_point_in_area/5(speed_min)
  range_min/1 -> sub_point_in_area/3(range_min)
  Add/1 -> sub_point_in_area/1(azimuth_min)
  Add1/1 -> sub_point_in_area/2(azimuth_max)
  azimuth_max/1 -> Add1/2
  azimuth_min/1 -> Add/1
  current_ego_wheel_angle/1 -> Add1/1, Add/2
  Constant/1 -> Divide/2
  Divide/1 -> Product/2
  Product/1 -> sub_point_in_area/4(range_max)
  range_savety_const/1 -> Product/1
  Bus_In/1 -> Bus Selector/1
  Bus Selector/1 -> sub_point_in_area/Enable  "<Radar_Mode>"
  Bus Selector/3 -> sub_point_in_area/11(u)  "<Radar_Punkt>"

== system D_20231120_Modell_Inbetriebnahme_BreakOutBox_Jetson/Read RC Control ==
  Bus_In : Inport
  1-D Lookup Table : Lookup_n-D  NumberOfTableDimensions=1  BreakpointsForDimension1=[0 50 100]  Table=[-1 0 1]  InternalRulePriority=Speed  RndMeth=Simplest
  Bus Selector : BusSelector  OutputSignals=IO691_Out.IO691_CAN_Sensoren.RC_Fahrpedal,IO691_Out.IO691_CAN_Sensoren.RC_Lenkung
  Compare To Constant : simulink/Logic and Bit Operations/Compare To Constant  relop===  const=255  OutDataTypeStr=boolean
  Compare To Constant1 : simulink/Logic and Bit Operations/Compare To Constant  relop===  const=255  OutDataTypeStr=boolean
  Constant : Constant  Value=50
  Constant1 : Constant  Value=50
  Constant2 : Constant  Value=100
  Divide : Product  Inputs=*/
  IC : InitialCondition  Value=0
  IC1 : InitialCondition  Value=0.5
  Saturation : Saturate  UpperLimit=100  LowerLimit=0
  Saturation1 : Saturate  UpperLimit=100  LowerLimit=0
  Switch : Switch  Criteria=u2 > Threshold  Threshold=0.5  SaturateOnIntegerOverflow=off  InputSameDT=off
  Switch1 : Switch  Criteria=u2 > Threshold  Threshold=0.5  SaturateOnIntegerOverflow=off  InputSameDT=off
  Transfer Fcn : TransferFcn  Denominator=[0.05 1]
  Transfer Fcn1 : TransferFcn  Denominator=[0.05 1]
  Lenkung : Outport
  Fahrpedal : Outport  Port=2
  wires:
  Bus Selector/2 -> Compare To Constant1/1, Switch1/3  "<RC_Lenkung>"
  Bus_In/1 -> Bus Selector/1
  Bus Selector/1 -> Compare To Constant/1, Switch/3  "<RC_Fahrpedal>"
  IC/1 -> Fahrpedal/1
  IC1/1 -> Lenkung/1
  Compare To Constant/1 -> Switch/2
  Constant/1 -> Switch/1
  Compare To Constant1/1 -> Switch1/2
  Constant1/1 -> Switch1/1
  Switch/1 -> Saturation/1
  Switch1/1 -> Saturation1/1
  Saturation/1 -> 1-D Lookup Table/1
  Saturation1/1 -> Divide/1
  Divide/1 -> Transfer Fcn1/1
  1-D Lookup Table/1 -> Transfer Fcn/1
  Constant2/1 -> Divide/2
  Transfer Fcn/1 -> IC/1
  Transfer Fcn1/1 -> IC1/1
